simulink model "bldc_trest53"  (Simulink 10.3)
settings: Solver=ode3  StartTime=0.0  StopTime=1.5  FixedStep=10e-6  RelTol=1e-3
undefined symbols (not defined in the file): B, J, K, L, P, R
libraries: simulink x6, spsVoltageMeasurementLib x6, spsSeriesRLCLoadLib x3, spspowerguiLib x1, spsDCVoltageSourceLib x1, spsThreePhaseParallelRLCBranchLib x1, spsUniversalBridgeLib x1
settings Model: Creator=SONY  LastModifiedBy=laxmi  MultithreadedSim=on
settings DataIOCC: SaveFormat=StructureWithTime  SignalLoggingSaveFormat=Dataset  ReturnWorkspaceOutputs=on
settings OptimizationCC: ExpressionDepthLimit=128
settings DebuggingCC: UnderspecifiedInitializationDetection=Simplified  MergeDetectMultiDrivingBlocksExec=error  FcnCallInpInsideContextMsg=error  StateNameClashWarn=none  SFUnexpectedBacktrackingDiag=error  SFNoUnconditionalDefaultTransitionDiag=error
settings HardwareCC: ProdBitPerPointer=64  ProdLargestAtomicFloat=Float  ProdIntDivRoundTo=Zero  ProdEndianess=LittleEndian  ProdHWDeviceType=Specified
settings ModelReferenceCC: PropagateSignalLabelsOutOfModel=on
settings SFSimCC: SimUseLocalCustomCode=on
settings RTWCC: RTWUseLocalCustomCode=on
settings GRTTargetCC: TargetLangStandard=C99 (ISO)  CombineOutputUpdateFcns=on  GRTInterface=off
settings ConfigComp: CovMetricSettings=dwe  CovSaveCumulativeToWorkspaceVar=off  CovSaveSingleToWorkspaceVar=off  CovExternalEMLEnable=on

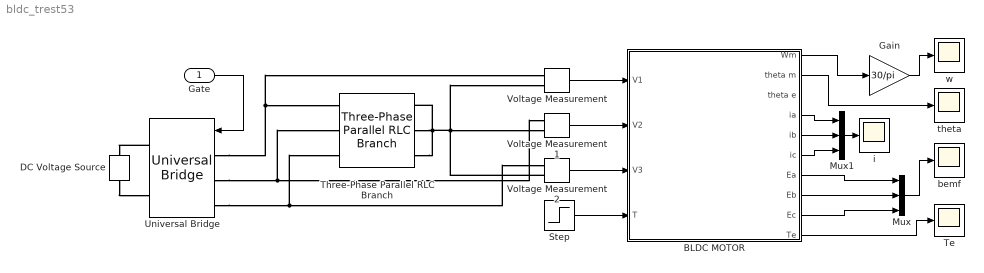
== system bldc_trest53 ==
  Gate : Inport
  BLDC MOTOR : Subsystem
  DC Voltage Source : spsDCVoltageSourceLib/DC Voltage Source  Amplitude=300  Measurements=None
  Gain : Gain  Gain=30/pi
  Mux : Mux  Inputs=3
  Mux1 : Mux  Inputs=3
  Step : Step  Time=0.5  After=9  SampleTime=0
  Te : Scope
  Three-Phase Parallel RLC Branch : spsThreePhaseParallelRLCBranchLib/Three-Phase Parallel RLC Branch  LConnTagsString=A|B|C  RConnTagsString=A|B|C  BranchType=R  Resistance=1  Inductance=1e-3  Capacitance=1e-6  Measurements=None
      settings: SourceProductBaseCode=PS
  Universal Bridge : spsUniversalBridgeLib/Universal Bridge  Arms=3  SnubberResistance=5000  SnubberCapacitance=1e-6  Device=MOSFET / Diodes  Ron=1e-3  Lon=0  ForwardVoltages="[  0  0  ]"  ForwardVoltage=0  GTOparameters=[ 10e-6 , 20e-6 ]  IGBTparameters=[ 1e-6 , 2e-6 ]  Measurements=None  Measurements_2=None  converterType=Rectifier
  Voltage Measurement : spsVoltageMeasurementLib/Voltage Measurement  PhasorSimulation=off  OutputType=Complex  PSBequivalent=0
  Voltage Measurement1 : spsVoltageMeasurementLib/Voltage Measurement  PhasorSimulation=off  OutputType=Complex  PSBequivalent=0
  Voltage Measurement2 : spsVoltageMeasurementLib/Voltage Measurement  PhasorSimulation=off  OutputType=Complex  PSBequivalent=0
  bemf : Scope
  i : Scope
  theta : Scope
  w : Scope
  wires:
  BLDC MOTOR/1(Wm) -> Gain/1
  BLDC MOTOR/2(theta m) -> theta/1
  BLDC MOTOR/4(ia) -> Mux1/1
  BLDC MOTOR/5(ib) -> Mux1/2
  BLDC MOTOR/6(ic) -> Mux1/3
  BLDC MOTOR/7(Ea) -> Mux/1
  BLDC MOTOR/8(Eb) -> Mux/2
  BLDC MOTOR/9(Ec) -> Mux/3
  BLDC MOTOR/10(Te) -> Te/1
  Step/1 -> BLDC MOTOR/4(T)
  Mux/1 -> bemf/1
  Mux1/1 -> i/1
  Gain/1 -> w/1
  Voltage Measurement2/1 -> BLDC MOTOR/3(V3)
  Voltage Measurement/1 -> BLDC MOTOR/1(V1)
  Voltage Measurement1/1 -> BLDC MOTOR/2(V2)
  Gate/1 -> Universal Bridge/1
  connections:
  Universal Bridge/RConn1 -- DC Voltage Source/RConn1
  DC Voltage Source/LConn1 -- Universal Bridge/RConn2
  Three-Phase Parallel RLC Branch/RConn2 -- Three-Phase Parallel RLC Branch/RConn1 -- Voltage Measurement/LConn2 -- Voltage Measurement2/LConn2 -- Voltage Measurement1/LConn2 -- Three-Phase Parallel RLC Branch/RConn3
  Universal Bridge/LConn1 -- Voltage Measurement/LConn1 -- Three-Phase Parallel RLC Branch/LConn1
  Universal Bridge/LConn2 -- Three-Phase Parallel RLC Branch/LConn2 -- Voltage Measurement1/LConn1
  Universal Bridge/LConn3 -- Voltage Measurement2/LConn1 -- Three-Phase Parallel RLC Branch/LConn3

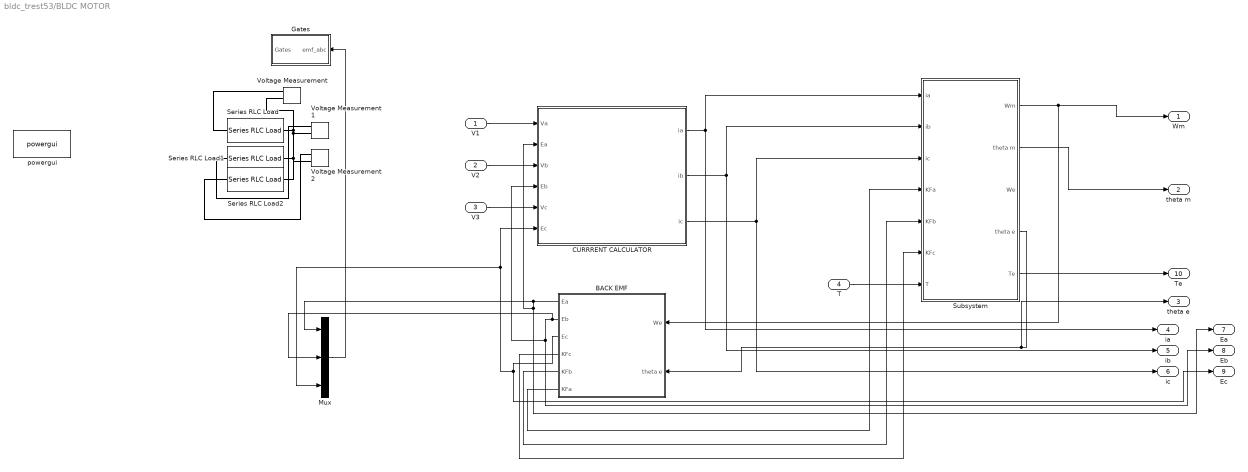
== system bldc_trest53/BLDC MOTOR ==
  V1 : Inport
  V2 : Inport  Port=2
  V3 : Inport  Port=3
  T : Inport  Port=4
  BACK EMF : Subsystem
  CURRRENT CALCULATOR : Subsystem
  Gates : Subsystem
  Mux : Mux  Inputs=3
  Series RLC Load : spsSeriesRLCLoadLib/Series RLC Load  LConnTagsString=a  RConnTagsString=__new0  NominalVoltage=1000  NominalFrequency=60  ActivePower=10e3  InductivePower=100  CapacitivePower=100  Setx0=off  InitialVoltage=0  SetiL0=off  InitialCurrent=0  Measurements=None  LoadType=constant Z
  Series RLC Load1 : spsSeriesRLCLoadLib/Series RLC Load  LConnTagsString=a  RConnTagsString=__new0  NominalVoltage=1000  NominalFrequency=60  ActivePower=10e3  InductivePower=100  CapacitivePower=100  Setx0=off  InitialVoltage=0  SetiL0=off  InitialCurrent=0  Measurements=None  LoadType=constant Z
  Series RLC Load2 : spsSeriesRLCLoadLib/Series RLC Load  LConnTagsString=a  RConnTagsString=__new0  NominalVoltage=1000  NominalFrequency=60  ActivePower=10e3  InductivePower=100  CapacitivePower=100  Setx0=off  InitialVoltage=0  SetiL0=off  InitialCurrent=0  Measurements=None  LoadType=constant Z
  Subsystem : Subsystem
  Voltage Measurement : spsVoltageMeasurementLib/Voltage Measurement  PhasorSimulation=off  OutputType=Complex  PSBequivalent=0
  Voltage Measurement1 : spsVoltageMeasurementLib/Voltage Measurement  PhasorSimulation=off  OutputType=Complex  PSBequivalent=0
  Voltage Measurement2 : spsVoltageMeasurementLib/Voltage Measurement  PhasorSimulation=off  OutputType=Complex  PSBequivalent=0
  powergui : spspowerguiLib/powergui  Priority=1  SimulationMode=Continuous  SampleTime=50e-6  frequency=60  Iterations=50  frequencyindice=0  Pbase=100e6  ErrMax=1e-4  UnitsV=kV  UnitsW=MW  buscounter=0  FunctionMessages=off  echomessages=off  EnableUseOfTLC=off  CurrentSourceSwitches=off  DisableSnubberDevices=off  DisableRonSwitches=off  DisableVfSwitches=off  DisplayEquations=off  AutomaticDiscreteSolvers=off  SolverType=Tustin/Backward Euler (TBE)  Interpol=off  ExternalGateDelay=off  methode=off  Ts=100  x0status=blocks  SPID=on  SwTol=0  HookPort=off  NonlinearTolerance=1e-4  nMaxIteration=100  ContinueOnMaxIteration=off  RestoreLinks=warning  ResistiveCurrentMeasurement=off  Frange=[0:2:500]  Ylog=off  Xlog=on  ShowGrid=off  save=off  variable=ZData  structure=0  ZoomFFT=off  StartTime=0.0  cycles=1  DisplayStyle=1  fundamental=60  FreqAxis=off  MaxFrequency=1000  frequencyindicesteady=1  RmsSteady=1  display=off
  Wm : Outport
  theta m : Outport  Port=2
  theta e : Outport  Port=3
  ia : Outport  Port=4
  ib : Outport  Port=5
  ic : Outport  Port=6
  Ea : Outport  Port=7
  Eb : Outport  Port=8
  Ec : Outport  Port=9
  Te : Outport  Port=10
  wires:
  CURRRENT CALCULATOR/1(ia) -> ia/1, Subsystem/1(ia)
  CURRRENT CALCULATOR/2(ib) -> ib/1, Subsystem/2(ib)
  CURRRENT CALCULATOR/3(ic) -> ic/1, Subsystem/3(ic)
  BACK EMF/1(Ea) -> Mux/1, Ea/1, CURRRENT CALCULATOR/2(Ea)
  BACK EMF/2(Eb) -> Mux/2, Eb/1, CURRRENT CALCULATOR/4(Eb)
  BACK EMF/3(Ec) -> Ec/1, Mux/3, CURRRENT CALCULATOR/6(Ec)
  Subsystem/4(theta e) -> BACK EMF/2(theta e), theta e/1
  BACK EMF/6(KFa) -> Subsystem/4(KFa)
  BACK EMF/5(KFb) -> Subsystem/5(KFb)
  BACK EMF/4(KFc) -> Subsystem/6(KFc)
  Subsystem/2(theta m) -> theta m/1
  Subsystem/5(Te) -> Te/1
  T/1 -> Subsystem/7(T)
  Subsystem/1(Wm) -> BACK EMF/1(We), Wm/1
  Mux/1 -> Gates/1("emf_abc ")
  V1/1 -> CURRRENT CALCULATOR/1(Va)
  V2/1 -> CURRRENT CALCULATOR/3(Vb)
  V3/1 -> CURRRENT CALCULATOR/5(Vc)
  connections:
  Voltage Measurement/LConn1 -- Series RLC Load/LConn1
  Voltage Measurement1/LConn1 -- Series RLC Load1/LConn1
  Voltage Measurement2/LConn1 -- Series RLC Load2/LConn1
  Series RLC Load/RConn1 -- Voltage Measurement/LConn2 -- Series RLC Load2/RConn1 -- Voltage Measurement2/LConn2 -- Series RLC Load1/RConn1 -- Voltage Measurement1/LConn2

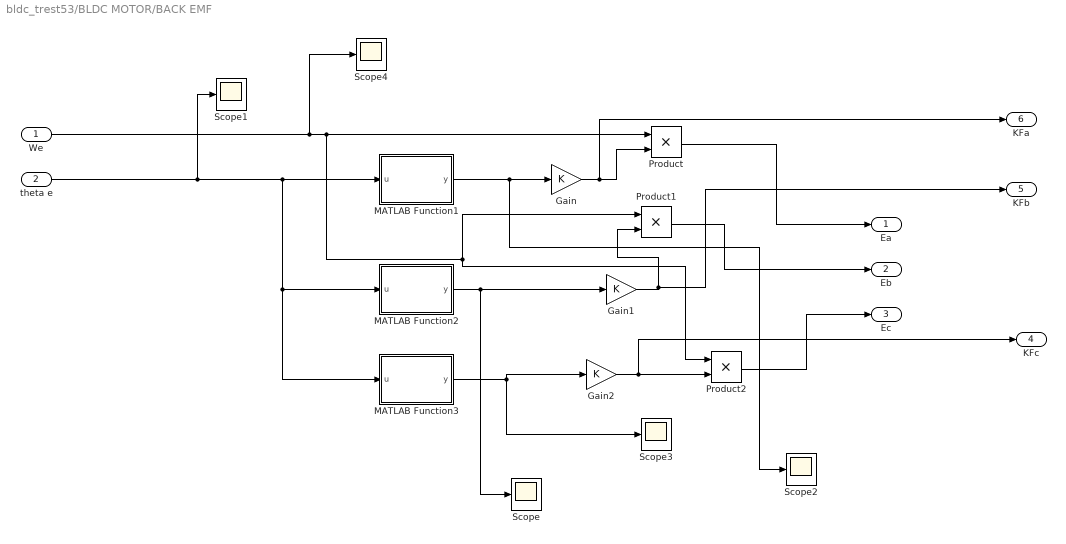
== system bldc_trest53/BLDC MOTOR/BACK EMF ==
  We : Inport
  theta e : Inport  Port=2
  Gain : Gain  Gain=K
  Gain1 : Gain  Gain=K
  Gain2 : Gain  Gain=K
  MATLAB Function1 : MATLAB Function  TreatAsAtomicUnit=on
  MATLAB Function2 : MATLAB Function  TreatAsAtomicUnit=on
  MATLAB Function3 : MATLAB Function  TreatAsAtomicUnit=on
  Product : Product
  Product1 : Product
  Product2 : Product
  Scope{,1..4} (5 alike) : Scope
  Ea : Outport
  Eb : Outport  Port=2
  Ec : Outport  Port=3
  KFc : Outport  Port=4
  KFb : Outport  Port=5
  KFa : Outport  Port=6
  wires:
  We/1 -> Scope4/1, Product1/1, Product2/1, Product/1
  Gain1/1 -> KFb/1, Product1/2
  MATLAB Function3/1(y) -> Scope3/1, Gain2/1
  Gain2/1 -> KFc/1, Product2/2
  MATLAB Function1/1(y) -> Scope2/1, Gain/1
  Gain/1 -> KFa/1, Product/2
  Product/1 -> Ea/1
  MATLAB Function2/1(y) -> Scope/1, Gain1/1
  Product1/1 -> Eb/1
  Product2/1 -> Ec/1
  theta e/1 -> MATLAB Function2/1(u), MATLAB Function3/1(u), MATLAB Function1/1(u), Scope1/1

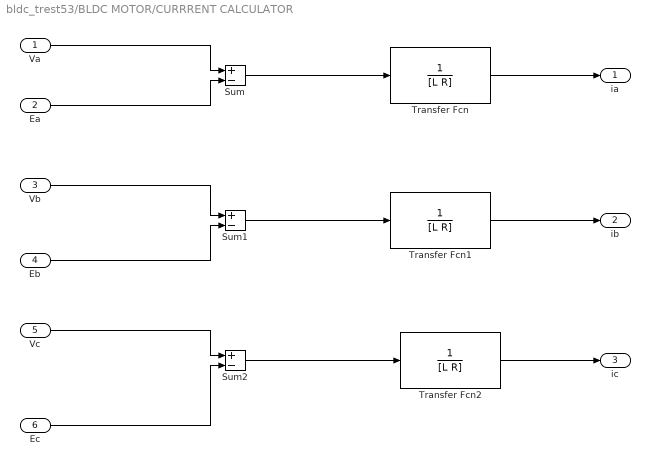
== system bldc_trest53/BLDC MOTOR/CURRRENT CALCULATOR ==
  Va : Inport
  Ea : Inport  Port=2
  Vb : Inport  Port=3
  Eb : Inport  Port=4
  Vc : Inport  Port=5
  Ec : Inport  Port=6
  Sum : Sum  Inputs=+-
  Sum1 : Sum  Inputs=+-
  Sum2 : Sum  Inputs=+-
  Transfer Fcn : TransferFcn  Denominator=[L R]
  Transfer Fcn1 : TransferFcn  Denominator=[L R]
  Transfer Fcn2 : TransferFcn  Denominator=[L R]
  ia : Outport
  ib : Outport  Port=2
  ic : Outport  Port=3
  wires:
  Eb/1 -> Sum1/2
  Vc/1 -> Sum2/1
  Sum/1 -> Transfer Fcn/1
  Sum2/1 -> Transfer Fcn2/1
  Sum1/1 -> Transfer Fcn1/1
  Vb/1 -> Sum1/1
  Ea/1 -> Sum/2
  Va/1 -> Sum/1
  Ec/1 -> Sum2/2
  Transfer Fcn/1 -> ia/1
  Transfer Fcn1/1 -> ib/1
  Transfer Fcn2/1 -> ic/1

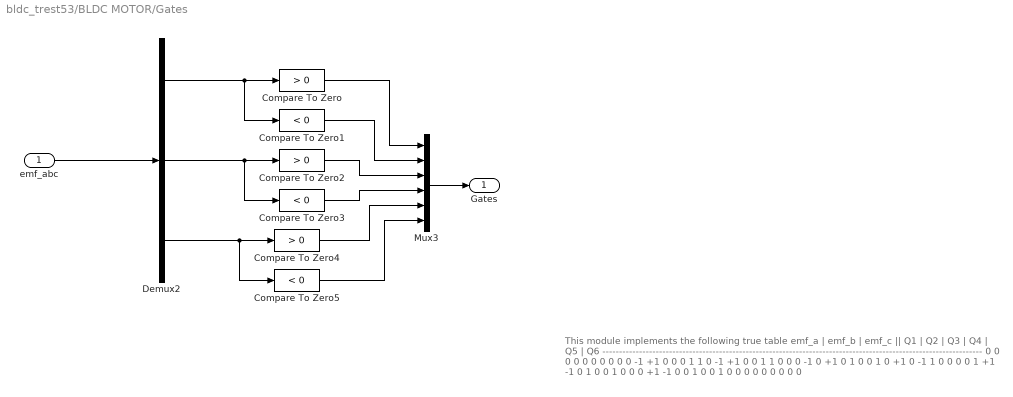
== system bldc_trest53/BLDC MOTOR/Gates ==
  note: This module implements the following true table
      |
      |    emf_a   |   emf_b   |   emf_c   ||   Q1   |   Q2   |   Q3   |   Q4   |   Q5   |   Q6
      |     ------------------------------------------------------------------------------------------------------------------
      |       0              0                0            0          0          0           0        0        0
      |       0               -1              +1          0          0          0           1        1        0
      |     -1              +1                0          0          1          1           0        0        0
      |     -1               0               +1          0          1         0           0        1        0
      |    +1               0                -1          1          0          0           0        0        1
      |    +1              -1                0           1          0          0           1        0        0
      |      0              +1               -1           0          0          1           0        0        1
      |     0              0                0             0          0          0           0        0        0
  "emf_abc " : Inport
  Compare To Zero : simulink/Logic and Bit Operations/Compare To Zero  relop=>  OutDataTypeStr=boolean  ZeroCross=off
  Compare To Zero1 : simulink/Logic and Bit Operations/Compare To Zero  relop=<  OutDataTypeStr=boolean  ZeroCross=off
  Compare To Zero2 : simulink/Logic and Bit Operations/Compare To Zero  relop=>  OutDataTypeStr=boolean  ZeroCross=off
  Compare To Zero3 : simulink/Logic and Bit Operations/Compare To Zero  relop=<  OutDataTypeStr=boolean  ZeroCross=off
  Compare To Zero4 : simulink/Logic and Bit Operations/Compare To Zero  relop=>  OutDataTypeStr=boolean  ZeroCross=off
  Compare To Zero5 : simulink/Logic and Bit Operations/Compare To Zero  relop=<  OutDataTypeStr=boolean  ZeroCross=off
  Demux2 : Demux  Outputs=3
  Mux3 : Mux  Inputs=6
  Gates : Outport
  wires:
  "emf_abc "/1 -> Demux2/1
  Mux3/1 -> Gates/1
  Demux2/1 -> Compare To Zero/1, Compare To Zero1/1
  Demux2/2 -> Compare To Zero2/1, Compare To Zero3/1
  Demux2/3 -> Compare To Zero4/1, Compare To Zero5/1
  Compare To Zero/1 -> Mux3/1
  Compare To Zero1/1 -> Mux3/2
  Compare To Zero2/1 -> Mux3/3
  Compare To Zero3/1 -> Mux3/4
  Compare To Zero4/1 -> Mux3/5
  Compare To Zero5/1 -> Mux3/6

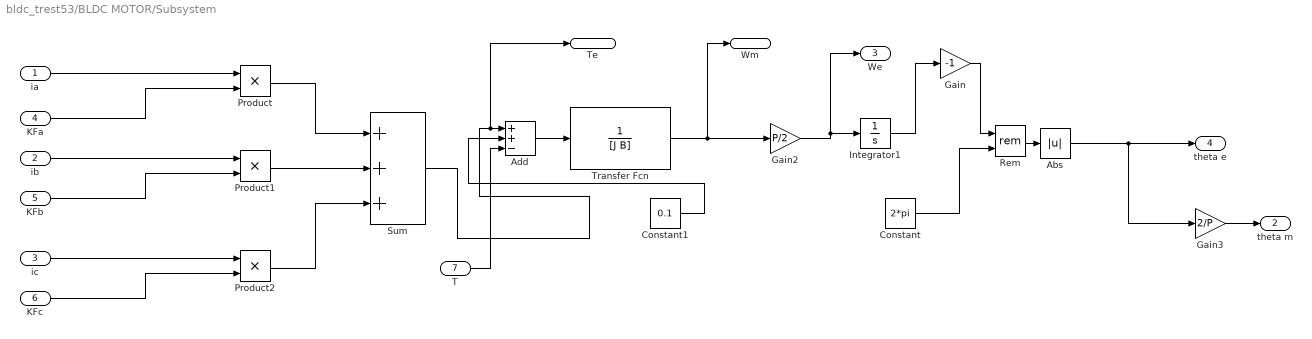
== system bldc_trest53/BLDC MOTOR/Subsystem ==
  ia : Inport
  ib : Inport  Port=2
  ic : Inport  Port=3
  KFa : Inport  Port=4
  KFb : Inport  Port=5
  KFc : Inport  Port=6
  T : Inport  Port=7
  Abs : Abs
  Add : Sum  Inputs=++-
  Constant : Constant  Value=2*pi
  Constant1 : Constant  Value=0.1
  Gain : Gain  Gain=-1
  Gain2 : Gain  Gain=P/2
  Gain3 : Gain  Gain=2/P
  Integrator1 : Integrator
  Product : Product
  Product1 : Product
  Product2 : Product
  Rem : Math  Operator=rem  SignedPower=on  SaturateOnIntegerOverflow=on
  Sum : Sum  Inputs=+++
  Transfer Fcn : TransferFcn  Denominator=[J B]
  Wm : Outport
  theta m : Outport  Port=2
  We : Outport  Port=3
  theta e : Outport  Port=4
  Te : Outport  Port=5
  wires:
  ia/1 -> Product/1
  ib/1 -> Product1/1
  ic/1 -> Product2/1
  KFb/1 -> Product1/2
  KFc/1 -> Product2/2
  Product/1 -> Sum/1
  Product1/1 -> Sum/2
  Product2/1 -> Sum/3
  KFa/1 -> Product/2
  T/1 -> Add/3
  Add/1 -> Transfer Fcn/1
  Gain2/1 -> Integrator1/1, We/1
  Gain3/1 -> theta m/1
  Constant/1 -> Rem/2
  Transfer Fcn/1 -> Gain2/1, Wm/1
  Sum/1 -> Te/1, Add/1
  Integrator1/1 -> Gain/1
  Gain/1 -> Rem/1
  Constant1/1 -> Add/2
  Rem/1 -> Abs/1
  Abs/1 -> Gain3/1, theta e/1

== matlab function BLDC MOTOR/BACK EMF/MATLAB Function1 ==
  data: u input double; y output double
function y = fcn(u)
%%codegen

if (0 <= u )&&(u < (pi)/6)
    u = 6*u/pi;
elseif ((pi)/6 <= u )&&(u < 5*pi/6)
    u = 1;
elseif (5*pi/6 <= u )&&(u < (7*pi)/6)
    u = -(6*u/pi)+6;
elseif ((7*pi)/6 <= u)&&(u  < 11*pi/6)
    u = -1;
elseif (11*pi/6 <= u )&&(u < 2*pi)
    u=(6*u/pi)-12;
end

y = u;

== matlab function BLDC MOTOR/BACK EMF/MATLAB Function2 ==
  data: u input double; y output double
function y = fcn(u)
%%codegen

if (0 <= u )&&(u < (pi)/2)
    u = -1;
elseif ((pi)/2 <= u)&&(u  < 5*pi/6)
    u = (6*u/pi)-4;
elseif (5*pi/6 <= u )&&(u < (9*pi)/6)
    u = 1;
elseif ((9*pi)/6 <= u )&&(u < 11*pi/6)
    u = -(6*u/pi)+10;
elseif (11*pi/6 <= u )&&(u < 2*pi)
    u= -1;
end

y = u;

== matlab function BLDC MOTOR/BACK EMF/MATLAB Function3 ==
  data: u input double; y output double
function y = fcn(u)
%%codegen

if (0 <= u )&&(u < (pi)/6)
    u = 1;
elseif ((pi)/6 <= u )&&(u < pi/2)
    u = -(6*u/pi)+2;
elseif (pi/2 <= u )&&(u < (7*pi)/6)
    u = -1;
elseif ((7*pi)/6 <= u )&&(u < 9*pi/6)
    u = (6*u/pi)-8;
elseif (9*pi/6 <= u )&&(u < 2*pi)
    u= 1;
end

y = u;
